simulink model "ORC_physical_modified"  (R2017a)
settings: Solver=VariableStepAuto  StartTime=0.0  StopTime=10.0  RelTol=1e-3
undefined symbols (not defined in the file): L_init, pipe_area, Throttle_param
libraries: fl_lib x16, nesl_utility x5, RankineCycle_lib x3
(part 5 of 5)

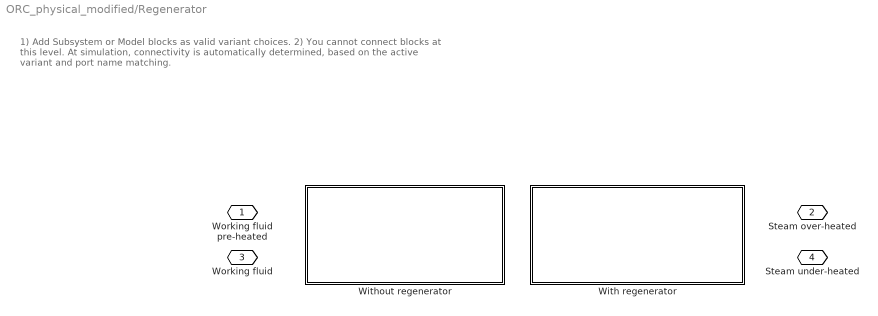
== system ORC_physical_modified/Regenerator ==
  note: 1) Add Subsystem or Model blocks as valid variant choices.
      | 2) You cannot connect blocks at this level. At simulation, connectivity is automatically
      | determined, based on the active variant and port name matching.
  With regenerator : Subsystem  VariantControl=Variant1
  Without regenerator : Subsystem  VariantControl=(default)
  " Working fluid pre-heated " : PMIOPort  Port=1  Side=Left
  Steam over-heated : PMIOPort  Port=2  Side=Right
  "Working fluid " : PMIOPort  Port=3  Side=Left
  " Steam under-heated  " : PMIOPort  Port=4  Side=Right

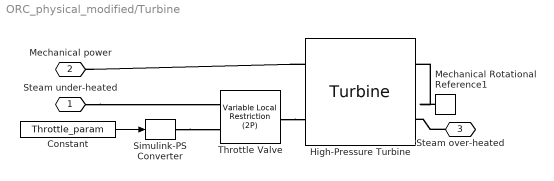
== system ORC_physical_modified/Turbine ==
  Constant : Constant  Value=Throttle_param
  High-Pressure Turbine : RankineCycle_lib/Turbine  p_A_nominal=3.5 MPa  p_B_nominal=1 MPa  mdot_nominal=1.5 kg/s  v_A_nominal=0.085 m^3/kg  isentropic_efficiency=0.9  mechanical_efficiency=0.9  area_A=pipe_area m^2  area_B=pipe_area m^2
  Mechanical Rotational Reference1 : fl_lib/Mechanical/Rotational Elements/Mechanical Rotational Reference
      settings: SourceProductName=Foundation Library
  Simulink-PS Converter : nesl_utility/Simulink-PS Converter  PhysicalDomain=network_engine_domain  SubClassName=ps_input  LeftPortType=input  RightPortType=output  PseudoPeriodic=off  Frequencies=[]  NoiseDistribution=none  NoiseParameters=[]  Unit=m^2  AffineConversion=off  FilteringAndDerivatives=provide  SimscapeFilterOrder=1  InputFilterTimeConstant=0.001  UdotUserProvided=0
  Throttle Valve : fl_lib/Two-Phase Fluid/Elements/Variable Local Restriction (2P)  min_area=1e-10 m^2  max_area=pipe_area / 10 m^2  area=pipe_area m^2  Cd=0.64  B_lam=0.999
      settings: SourceProductName=Foundation Library
  Steam under-heated : PMIOPort  Port=1  Side=Left
  Mechanical power : PMIOPort  Port=2  Side=Right
  Steam over-heated : PMIOPort  Port=3  Side=Right
  wires:
  Constant/1 -> Simulink-PS Converter/1
  connections:
  Mechanical Rotational Reference1/LConn1 -- High-Pressure Turbine/RConn2
  High-Pressure Turbine/LConn2 -- Mechanical power/RConn1
  Steam over-heated/RConn1 -- High-Pressure Turbine/RConn1
  Throttle Valve/RConn1 -- High-Pressure Turbine/LConn1
  Steam under-heated/RConn1 -- Throttle Valve/LConn1
  Simulink-PS Converter/RConn1 -- Throttle Valve/LConn2

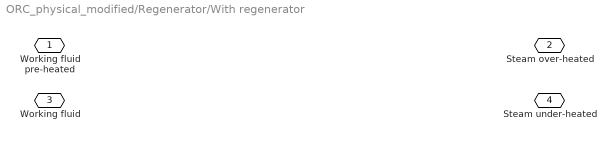
== system ORC_physical_modified/Regenerator/With regenerator ==
  " Working fluid pre-heated " : PMIOPort  Port=1  Side=Left
  Steam over-heated : PMIOPort  Port=2  Side=Right
  "Working fluid " : PMIOPort  Port=3  Side=Left
  " Steam under-heated  " : PMIOPort  Port=4  Side=Right

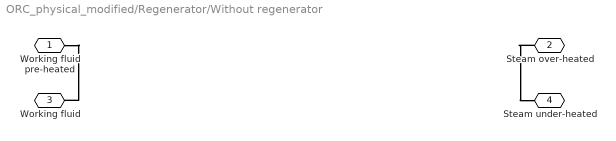
== system ORC_physical_modified/Regenerator/Without regenerator ==
  " Working fluid pre-heated " : PMIOPort  Port=1  Side=Left
  Steam over-heated : PMIOPort  Port=2  Side=Right
  "Working fluid " : PMIOPort  Port=3  Side=Left
  " Steam under-heated  " : PMIOPort  Port=4  Side=Right
  connections:
  " Working fluid pre-heated "/RConn1 -- "Working fluid "/RConn1
  Steam over-heated/RConn1 -- " Steam under-heated  "/RConn1
